simulink model "cubesat_propagation"  (R2019b)
settings: Solver=FixedStepAuto  StartTime=0.0  StopTime=10000  FixedStep=dT  RelTol=1e-5
PostLoadFcn:
  | if builtin('license','test','Virtual_Reality_Toolbox')
  |     set_param([bdroot(gcs) '/Simulink 3D Animation'], 'enableVis', 'on')
  | else
  |     set_param([bdroot(gcs) '/Simulink 3D Animation'], 'enableVis', 'off')
  | end
InitFcn:
  | if strcmp(get_param([bdroot(gcs) '/Simulink 3D Animation'], 'enableVis'), 'on')
  |     if ~builtin('license','checkout','Virtual_Reality_Toolbox')
  |         error(message('aeroblks_cubesat:cubesat:licenseFailAnimTemplate'));
  |     end
  | end
model workspace (MATLAB code in the model file + MAT data in the model file):
  aeroCoeff : object (value not decoded)
  environment : EarthRefAlt (value not decoded)
  initCond : object (value not decoded)
  inputs0 : object (value not decoded)
  states0 : object (value not decoded)
  vehicle : object (value not decoded)
  other statements: initialize6DOFSkyHogg;
values from neighbouring files (symbols this model uses):
  a = input("Semimajor axis [km]: ")    [SCARSSetup.m]    (also in pwsat2_setup.m = 6960989.91401; pwsat2_tle.m = 6960989.91401; scars_setup.m = 7378000; startup.m = 8000000)
  e = input("Eccentricity [-]: ")    [SCARSSetup.m]    (also in pwsat2_setup.m = 0.0011871; pwsat2_tle.m = 0.0011871; scars_setup.m = 0; startup.m = 0)
  incl = input("Inclination [deg]: ")    [SCARSSetup.m]    (also in pwsat2_setup.m = deg2rad(97.7672); pwsat2_tle.m = deg2rad(97.7672); scars_setup.m = deg2rad(0.00001); startup.m = deg2rad(45))
  initEuler = [0 0 0]    [SCARSSetup.m]    (also in pwsat2_setup.m; scars_setup.m)
  initEulerRates = [0.0 0.0 0.0]    [SCARSSetup.m]    (also in pwsat2_setup.m = -scars_out.omega_b(end,:); scars_setup.m = [0 0 0])
  julian = juliandate(utc)    [SCARSSetup.m]    (also in pwsat2_setup.m; pwsat2_tle.m; scars_setup.m)
  RA = input("Right ascension of the ascending node [deg]: ")    [SCARSSetup.m]    (also in pwsat2_setup.m = deg2rad(56.1804); pwsat2_tle.m = deg2rad(56.1804); scars_setup.m = deg2rad(0); startup.m = deg2rad(90))
  s = ecc * sinh(eanom)    [kepler1.m]
  TA = deg2rad(0)    [scars_setup.m]    (also in startup.m; startup_cubesat_ref.m = deg2rad(302.9234))
  w = input("Argument of periapsis [deg]: ")    [SCARSSetup.m]    (also in pwsat2_setup.m = deg2rad(236.0402); pwsat2_tle.m = deg2rad(236.0402); scars_setup.m = deg2rad(0); startup.m = deg2rad(0))
undefined symbols (not defined in the file or in its folder): constraintAxes, Earth, euler0, km, pointing, pqr0, WGS84
libraries: aerolibutil x13, aerolibconvert2 x5, sharedtransform x3, asbCubeSatBlockLib x2, simulink x2, aerolibcelestial x2, aerolib6dof2 x1, aerolibtransform2 x1, sharedutil x1, aerolibobsolete x1, vrlib x1, aerolibgravity2 x1
(part 2 of 2)

== system cubesat_propagation/CubeSat Vehicle/First Constraint/Standby ==
  Action Port : ActionPort  ActionPortLabel=default:
  Constant : Constant  Value=[0 0 0]'  OutDataTypeStr=Inherit: Inherit via back propagation
  O : Outport  VectorParamsAs1DForOutWhenUnconnected=off
  wires:
  Constant/1 -> O/1

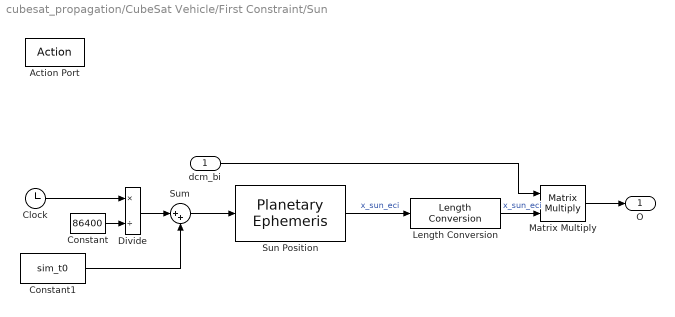
== system cubesat_propagation/CubeSat Vehicle/First Constraint/Sun  ==
  dcm_bi : Inport
  Action Port : ActionPort  ActionPortLabel=case [ 2 ]:
  Clock : Clock
  Constant : Constant  Value=86400
  Constant1 : Constant  RequirementInfo={} %GIDa_3340d8fb_5b7e_4e83_88e1_92a85cc7add9  Value=sim_t0
  Divide : Product  Inputs=*/
  Length Conversion : aerolibconvert2/Length Conversion  IU=km  OU=m
  Matrix Multiply : Product  Multiplication=Matrix(*)
  Sum : Sum  Inputs=|++
  Sun Position : aerolibcelestial/Planetary Ephemeris  kmflag=km,km/s  epochflag=Julian date  de=DE421  nCenter=Earth  nTarget=Sun  errorflag=Error  velflag=off
      settings: SourceProductName=Aerospace Blockset  SourceProductBaseCode=AE
  O : Outport  VectorParamsAs1DForOutWhenUnconnected=off
  wires:
  Matrix Multiply/1 -> O/1
  Length Conversion/1 -> Matrix Multiply/2  "x_sun_eci"
  Divide/1 -> Sum/1
  Constant/1 -> Divide/2
  Sun Position/1 -> Length Conversion/1  "x_sun_eci"
  Clock/1 -> Divide/1
  Sum/1 -> Sun Position/1
  Constant1/1 -> Sum/2
  dcm_bi/1 -> Matrix Multiply/1

== system cubesat_propagation/Simulink 3D Animation/Antenna Position to VRML/ECEF to VRML ==
  M : Inport  PortDimensions=3
  Demux : Demux  Outputs=3
  Gain3 : Gain  Gain=-1
  Mux : Mux  Inputs=3
  VR : Outport  PortDimensions=3  VectorParamsAs1DForOutWhenUnconnected=off
  wires:
  M/1 -> Demux/1
  Demux/1 -> Gain3/1
  Demux/2 -> Mux/3
  Demux/3 -> Mux/2
  Mux/1 -> VR/1
  Gain3/1 -> Mux/1

== system cubesat_propagation/Simulink 3D Animation/Compute Earth Rotation Rate/Quaternion to VRML ==
  q : Inport
  Demux : Demux
  Gain : Gain  Gain=2
  Gain3 : Gain  Gain=[-1 1 1 1]
  Mux : Mux
  Selector : Selector  InputPortWidth=4  IndexOptions=Index vector (dialog)  Indices=[2 4 3 1]  OutputSizes=1
  Trigonometric Function : Trigonometry  Operator=acos
  AxisAngle : Outport  VectorParamsAs1DForOutWhenUnconnected=off
  wires:
  Demux/1 -> Trigonometric Function/1
  Trigonometric Function/1 -> Gain/1
  Mux/1 -> Selector/1
  q/1 -> Demux/1
  Gain3/1 -> AxisAngle/1
  Selector/1 -> Gain3/1
  Gain/1 -> Mux/1
  Demux/2 -> Mux/2
  Demux/3 -> Mux/3
  Demux/4 -> Mux/4

== system cubesat_propagation/Simulink 3D Animation/Compute Umbra Translation/unitVec ==
  I : Inport
  Divide : Product  Inputs=*/
  Dot Product : DotProduct  InputSameDT=on  OutDataTypeStr=Inherit: Inherit via internal rule
  Sqrt : Sqrt  SaturateOnIntegerOverflow=on
  O : Outport  VectorParamsAs1DForOutWhenUnconnected=off
  wires:
  Dot Product/1 -> Sqrt/1
  I/1 -> Divide/1, Dot Product/1, Dot Product/2
  Divide/1 -> O/1
  Sqrt/1 -> Divide/2

== system cubesat_propagation/Simulink 3D Animation/Sat Position to VRML/ECEF to VRML ==
  M : Inport  PortDimensions=3
  Demux : Demux  Outputs=3
  Gain3 : Gain  Gain=-1
  Mux : Mux  Inputs=3
  VR : Outport  PortDimensions=3  VectorParamsAs1DForOutWhenUnconnected=off
  wires:
  M/1 -> Demux/1
  Demux/1 -> Gain3/1
  Demux/2 -> Mux/3
  Demux/3 -> Mux/2
  Mux/1 -> VR/1
  Gain3/1 -> Mux/1

== system cubesat_propagation/Simulink 3D Animation/Sun Position to VRML/ECEF to VRML ==
  M : Inport  PortDimensions=3
  Demux : Demux  Outputs=3
  Gain3 : Gain  Gain=-1
  Mux : Mux  Inputs=3
  VR : Outport  PortDimensions=3  VectorParamsAs1DForOutWhenUnconnected=off
  wires:
  M/1 -> Demux/1
  Demux/1 -> Gain3/1
  Demux/2 -> Mux/3
  Demux/3 -> Mux/2
  Mux/1 -> VR/1
  Gain3/1 -> Mux/1
